simulink model "DC_Microgrid_Sim"  (R2023b)
settings: Solver=VariableStepDiscrete  StartTime=0.0  StopTime=72  MaxStep=1e-2  RelTol=1e-3
undefined symbols (not defined in the file or in its folder): dEgdT, EgRef, gcbh, Ion, k1, Lithium, Rsh_array5pc, sps_rtmsupport, Tref_K, Tsf, VT_ref
libraries: spsSeriesRLCBranchLib x7, spsVoltageMeasurementLib x5, SignalEditorBlockLib x2, spsCurrentMeasurementLib x2, spsDiodeLib x2, spsFirstOrderFilterLib x2, spsControlledCurrentSourceLib x2, spsPVarrayModel x2, spsBatteryLib x1, spsVariableResistorLib x1, spsBoostConverterLib x1, spsStairGeneratorLib x1
(part 9 of 9)

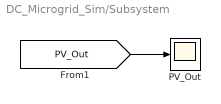
== system DC_Microgrid_Sim/Subsystem ==
  PV_Out : Scope
  wires:
  [PV_Out] -> PV_Out/1

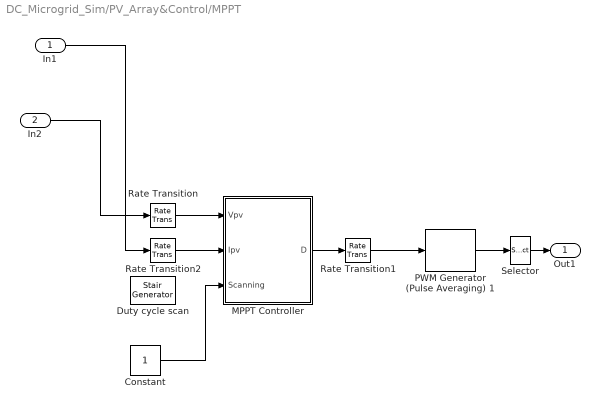
== system DC_Microgrid_Sim/PV_Array&Control/MPPT ==
  In1 : Inport
  In2 : Inport  Port=2
  Constant : Constant
  Duty cycle scan : spsStairGeneratorLib/Stair Generator  t=[0,0.40, 0.41]  e=[0, 1, 0]  Ts=2.5e-05
  MPPT Controller : Subsystem  mask(MPPT Controller - Perturb and Observe algorithm (PandO)){Dinit=0.39, Dlimits=[0.85, 0.30], deltaD=50e-6, Fc=1000, ScanDuration=0.25, Ts=2.5e-05}
      mask prompts: Dinit "Duty cycle (D) initial value"; Dlimits "D limits [Upper, Lower]"; deltaD "Increment value for PandO algorithm"; Fc "Measurement filter cutoff frequency (Hz)"; ScanDuration "Scanning mode duration (s)"; Ts "Sample time (s)"
      mask init:
      | Dmax=Dlimits(1);
      | Dmin=Dlimits(2);
      | SampleTime=Ts;
      | DeltaD_Scan=(Dmax-Dmin)*Ts/ScanDuration;
  PWM Generator (Pulse Averaging) 1 : spsPWMGeneratorPulseAveragingLib/PWM Generator (Pulse Averaging)  GeneratorType=Two-quadrant  Fc=20e3  InitialPhase=90  Ts=5e-06
  Rate Transition : RateTransition  OutPortSampleTime=2.5e-05
  Rate Transition1 : RateTransition  OutPortSampleTime=5e-06
  Rate Transition2 : RateTransition  OutPortSampleTime=2.5e-05
  Selector : Selector  InputPortWidth=2  IndexOptions=Index vector (dialog)  Indices=1  OutputSizes=1
  Out1 : Outport
  wires:
  Selector/1 -> Out1/1
  Rate Transition2/1 -> MPPT Controller/2(Ipv)
  In1/1 -> Rate Transition2/1
  In2/1 -> Rate Transition/1
  Rate Transition1/1 -> PWM Generator (Pulse Averaging) 1/1
  MPPT Controller/1(D) -> Rate Transition1/1
  Rate Transition/1 -> MPPT Controller/1(Vpv)
  PWM Generator (Pulse Averaging) 1/1 -> Selector/1
  Constant/1 -> MPPT Controller/3(Scanning)

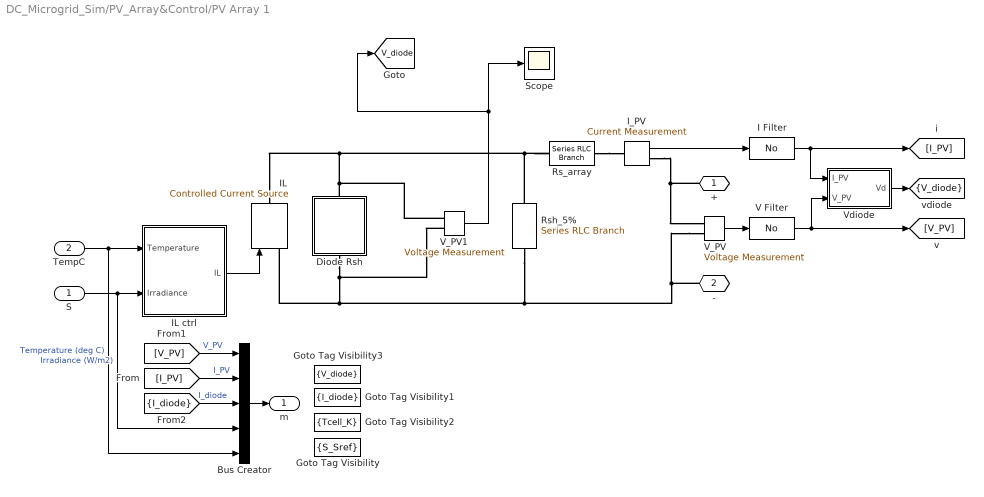
== system DC_Microgrid_Sim/PV_Array&Control/PV Array 1 ==
  S : Inport
  TempC : Inport  Port=2
  Bus Creator : BusCreator  Inputs=5
  Diode Rsh : Subsystem  AncestorBlock=spsPVarrayModel/Discrete Diode Rsh BAL
      mask Display:
      | plot(-75,-50,100,150, [-15 -15 43 -15 -15 -75],[50 8 50 92 50 50], ...
      |     [43 43],[8 94],[100 43], [50 50])
  Goto Tag Visibility : GotoTagVisibility  GotoTag=S_Sref
  Goto Tag Visibility1 : GotoTagVisibility  GotoTag=I_diode
  Goto Tag Visibility2 : GotoTagVisibility  GotoTag=Tcell_K
  Goto Tag Visibility3 : GotoTagVisibility  GotoTag=V_diode
  I Filter : spsPVarrayModel/No  SystemSampleTime=-1  VariantControl=Variant1  VariantActivationTime=update diagram  AllowFlexibleInterface=on  Latency=0  AutoFrameSizeCalculation=off
  IL : spsControlledCurrentSourceLib/Controlled Current Source  Initialize=on  Source_Type=AC  Amplitude=0  Phase=0  Frequency=0  Measurements=None
  IL ctrl : Subsystem
  I_PV : spsCurrentMeasurementLib/Current Measurement  PhasorSimulation=off  OutputType=Complex  PSBequivalent=0
  Rs_array : spsSeriesRLCBranchLib/Series RLC Branch  LConnTagsString=__new0  RConnTagsString=__new0  BranchType=R  Resistance=Rs*Nser/Npar  Inductance=1e-3  SetiL0=off  InitialCurrent=0  Capacitance=1e-6  Setx0=off  InitialVoltage=0  Measurements=None
  Rsh_5% : spsSeriesRLCBranchLib/Series RLC Branch  LConnTagsString=__new0  RConnTagsString=__new0  BranchType=R  Resistance=Rsh_array5pc  Inductance=1e-3  SetiL0=off  InitialCurrent=0  Capacitance=1e-6  Setx0=off  InitialVoltage=0  Measurements=None
  Scope : Scope
  V Filter : spsPVarrayModel/No  SystemSampleTime=-1  VariantControl=Variant1  VariantActivationTime=update diagram  AllowFlexibleInterface=on  Latency=0  AutoFrameSizeCalculation=off
  V_PV : spsVoltageMeasurementLib/Voltage Measurement  PhasorSimulation=off  OutputType=Complex  PSBequivalent=0
  V_PV1 : spsVoltageMeasurementLib/Voltage Measurement  PhasorSimulation=off  OutputType=Complex  PSBequivalent=0
  Vdiode : Subsystem
  + : PMIOPort  Side=Right
  - : PMIOPort  Port=2  Side=Right
  m : Outport  VectorParamsAs1DForOutWhenUnconnected=off
  tag scope: V_diode=global, V_diode=scoped
  wires:
  TempC/1 -> Bus Creator/5, IL ctrl/1(Temperature)  "Temperature (deg C)"
  S/1 -> IL ctrl/2(Irradiance), Bus Creator/4  "Irradiance (W/m2)"
  I_PV/1 -> I Filter/1
  Bus Creator/1 -> m/1
  IL ctrl/1(IL) -> IL/1
  V_PV/1 -> V Filter/1
  I Filter/1 -> Vdiode/1(I_PV), [I_PV]
  V Filter/1 -> [V_PV], Vdiode/2(V_PV)
  [I_PV] -> Bus Creator/2  "I_PV"
  [V_PV] -> Bus Creator/1  "V_PV"
  [I_diode] -> Bus Creator/3  "I_diode"
  Vdiode/1(Vd) -> [V_diode]
  V_PV1/1 -> [V_diode], Scope/1
  connections:
  +/RConn1 -- I_PV/RConn1 -- V_PV/LConn1
  Rs_array/LConn1 -- V_PV1/LConn1 -- Diode Rsh/LConn1 -- IL/RConn1 -- Rsh_5%/LConn1
  V_PV/LConn2 -- V_PV1/LConn2 -- Diode Rsh/RConn1 -- IL/LConn1 -- Rsh_5%/RConn1 -- -/RConn1
  Rs_array/RConn1 -- I_PV/LConn1

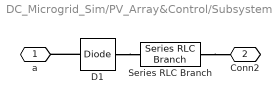
== system DC_Microgrid_Sim/PV_Array&Control/Subsystem ==
  D1 : spsDiodeLib/Diode  Ron=1e-3  Lon=0  Vf=.6  IC=0  UseSnubber=0  Rs=1e6  Cs=inf  Measurements=off
  Series RLC Branch : spsSeriesRLCBranchLib/Series RLC Branch  LConnTagsString=__new0  RConnTagsString=__new0  BranchType=RL  Resistance=20e-3  Inductance=20e-3  SetiL0=off  InitialCurrent=0  Capacitance=1e-6  Setx0=off  InitialVoltage=0  Measurements=None
  a : PMIOPort  Side=Left
  Conn2 : PMIOPort  Port=2  Side=Right
  connections:
  D1/LConn1 -- a/RConn1
  Series RLC Branch/RConn1 -- Conn2/RConn1
  D1/RConn1 -- Series RLC Branch/LConn1

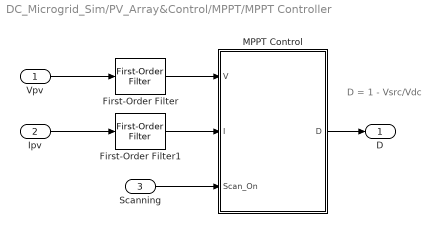
== system DC_Microgrid_Sim/PV_Array&Control/MPPT/MPPT Controller ==
  note: D = 1 - Vsrc/Vdc
  Vpv : Inport
  Ipv : Inport  Port=2
  Scanning : Inport  Port=3  PortDimensions=1
  First-Order Filter : spsFirstOrderFilterLib/First-Order Filter  FilterType=Lowpass  Tc=1/Fc  Ts=Ts  Initialize=off  Vac_Init=[0, 0, 60]  Vdc_Init=0  PlotResponse=off  FreqRange="[0,  200,  1]"
  First-Order Filter1 : spsFirstOrderFilterLib/First-Order Filter  FilterType=Lowpass  Tc=1/Fc  Ts=Ts  Initialize=off  Vac_Init=[0, 0, 60]  Vdc_Init=0  PlotResponse=off  FreqRange="[0,  200,  1]"
  MPPT Control : MATLAB Function  TreatAsAtomicUnit=on
  D : Outport  OutDataTypeStr=double  PortDimensions=1  VectorParamsAs1DForOutWhenUnconnected=off
  wires:
  First-Order Filter1/1 -> MPPT Control/2(I)
  First-Order Filter/1 -> MPPT Control/1(V)
  Ipv/1 -> First-Order Filter1/1
  Vpv/1 -> First-Order Filter/1
  MPPT Control/1(D) -> D/1
  Scanning/1 -> MPPT Control/3(Scan_On)

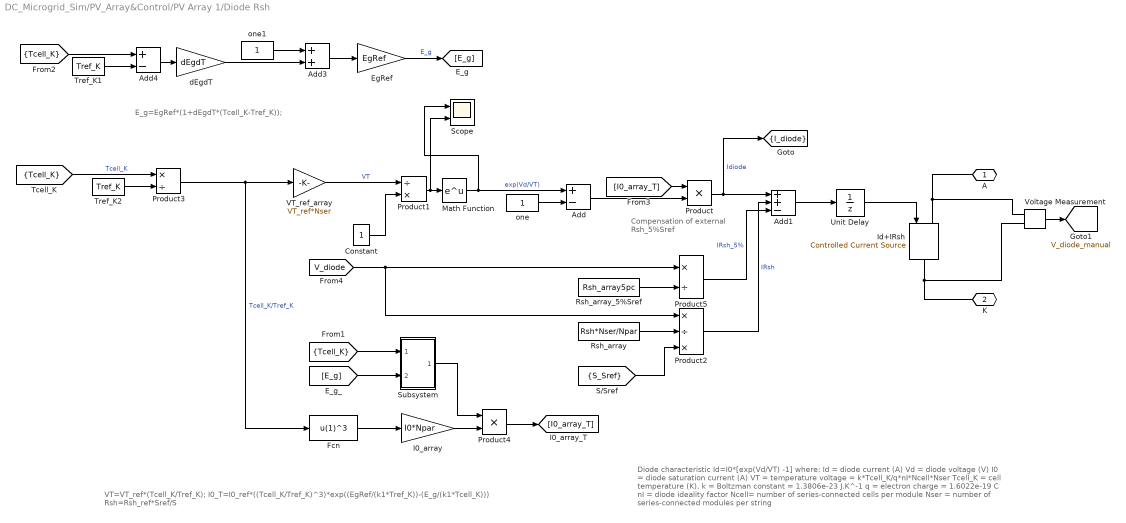
== system DC_Microgrid_Sim/PV_Array&Control/PV Array 1/Diode Rsh ==
  note: E_g=EgRef*(1+dEgdT*(Tcell_K-Tref_K));
  note: VT=VT_ref*(Tcell_K/Tref_K);
      | I0_T=I0_ref*((Tcell_K/Tref_K)^3)*exp((EgRef/(k1*Tref_K))-(E_g/(k1*Tcell_K)))
      | Rsh=Rsh_ref*Sref/S
  note: Diode characteristic
      |    Id=I0*[exp(Vd/VT) -1]
      |
      | where:
      |      Id = diode current (A)
      |      Vd = diode voltage (V)
      |      I0 = diode saturation current (A)
      |      VT = temperature voltage = k*Tcell_K/q*nI*Ncell*Nser
      | Tcell_K = cell temperature (K),
      |       k = Boltzman constant = 1.3806e-23 J.K^-1
      |       q = electron charge = 1.6022e-19 C
      |      nI = diode ideality factor
      |    Ncell= number of series-connected cells per module
      |    Nser = number of series-connected modules per string
  note: Compensation of
      | external Rsh_5%Sref
  Add : Sum  Inputs=+-
  Add1 : Sum  Inputs=++-
  Add3 : Sum
  Add4 : Sum  Inputs=+-
  Constant : Constant
  EgRef : Gain  Gain=EgRef
  Fcn : Fcn  Expr=u(1)^3
  I0_array : Gain  Gain=I0*Npar
  Id+IRsh : spsControlledCurrentSourceLib/Controlled Current Source  Initialize=on  Source_Type=AC  Amplitude=0  Phase=0  Frequency=0  Measurements=None
  Math Function : Math  SignedPower=on
  Product : Product  RndMeth=Zero
  Product1 : Product  Inputs=/*  RndMeth=Zero
  Product2 : Product  Inputs=*/*  RndMeth=Zero
  Product3 : Product  Inputs=*/  RndMeth=Zero
  Product4 : Product  Inputs=**  RndMeth=Zero
  Product5 : Product  Inputs=*/  RndMeth=Zero
  Rsh_array : Constant  Value=Rsh*Nser/Npar
  Rsh_array_5%Sref : Constant  Value=Rsh_array5pc
  Scope : Scope  NumInputPorts=2
  Subsystem : Subsystem
  Tref_K1 : Constant  Value=Tref_K
  Tref_K2 : Constant  Value=Tref_K
  Unit Delay : UnitDelay  SampleTime=Tsf  HasFrameUpgradeWarning=on
  VT_ref_array : Gain  Gain=VT_ref*Nser
  Voltage Measurement : spsVoltageMeasurementLib/Voltage Measurement  PhasorSimulation=off  OutputType=Complex  PSBequivalent=0
  dEgdT : Gain  Gain=dEgdT
  one : Constant
  one1 : Constant
  A : PMIOPort  Side=Left
  K : PMIOPort  Port=2  Side=Right
  tag scope: I_diode=scoped, V_diode_manual=global
  wires:
  [V_diode] -> Product2/1, Product5/1
  [S_Sref] -> Product2/3
  [I0_array_T] -> Product/1
  VT_ref_array/1 -> Product1/1  "VT"
  Add/1 -> Product/2
  Product4/1 -> [I0_array_T]
  Tref_K2/1 -> Product3/2
  [E_g] -> Subsystem/2(E_g)
  [Tcell_K] -> Subsystem/1(Tcell_K)
  Subsystem/1(exp) -> Product4/1
  Tref_K1/1 -> Add4/2
  [Tcell_K] -> Add4/1
  Fcn/1 -> I0_array/1
  I0_array/1 -> Product4/2
  EgRef/1 -> [E_g]  "E_g"
  Add3/1 -> EgRef/1
  dEgdT/1 -> Add3/2
  Add4/1 -> dEgdT/1
  one1/1 -> Add3/1
  Product3/1 -> Fcn/1, VT_ref_array/1  "Tcell_K/Tref_K"
  [Tcell_K] -> Product3/1  "Tcell_K"
  Rsh_array/1 -> Product2/2
  one/1 -> Add/2
  Product1/1 -> Scope/2, Math Function/1
  Product/1 -> [I_diode], Add1/1  "Idiode"
  Product2/1 -> Add1/2  "IRsh"
  Math Function/1 -> Scope/1, Add/1  "exp(Vd/VT)"
  Rsh_array_5%Sref/1 -> Product5/2
  Product5/1 -> Add1/3  "IRsh_5%"
  Add1/1 -> Unit Delay/1
  Unit Delay/1 -> Id+IRsh/1
  Voltage Measurement/1 -> [V_diode_manual]
  Constant/1 -> Product1/2
  connections:
  A/RConn1 -- Id+IRsh/LConn1 -- Voltage Measurement/LConn1
  Id+IRsh/RConn1 -- Voltage Measurement/LConn2 -- K/RConn1

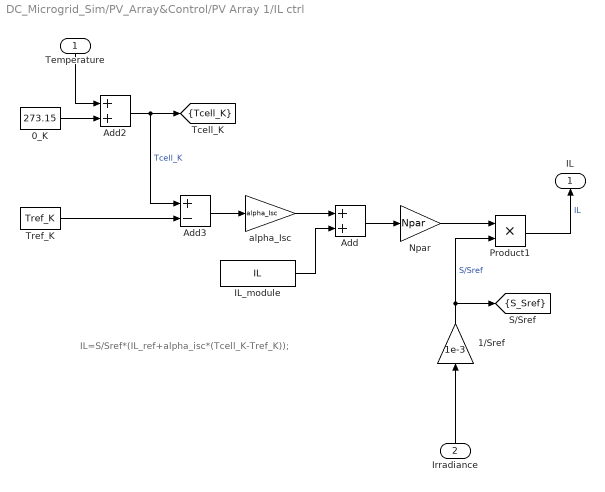
== system DC_Microgrid_Sim/PV_Array&Control/PV Array 1/IL ctrl ==
  note: IL=S/Sref*(IL_ref+alpha_isc*(Tcell_K-Tref_K));
  Temperature : Inport
  Irradiance : Inport  Port=2
  0_K : Constant  Value=273.15
  1/Sref : Gain  Gain=1e-3
  Add : Sum
  Add2 : Sum
  Add3 : Sum  Inputs=+-
  IL_module : Constant  Value=IL
  Npar : Gain  Gain=Npar
  Product1 : Product  Inputs=**  RndMeth=Zero
  Tref_K : Constant  Value=Tref_K
  alpha_Isc : Gain  Gain=alpha_Isc
  IL : Outport  VectorParamsAs1DForOutWhenUnconnected=off
  tag scope: S_Sref=scoped, Tcell_K=scoped
  wires:
  1/Sref/1 -> [S_Sref], Product1/2  "S/Sref"
  Npar/1 -> Product1/1
  Add2/1 -> [Tcell_K], Add3/1  "Tcell_K"
  Add/1 -> Npar/1
  0_K/1 -> Add2/2
  IL_module/1 -> Add/2
  Product1/1 -> IL/1  "IL"
  Tref_K/1 -> Add3/2
  Add3/1 -> alpha_Isc/1
  alpha_Isc/1 -> Add/1
  Irradiance/1 -> 1/Sref/1
  Temperature/1 -> Add2/1

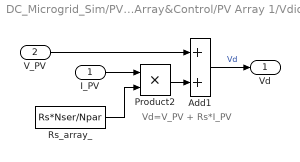
== system DC_Microgrid_Sim/PV_Array&Control/PV Array 1/Vdiode ==
  note: Vd=V_PV + Rs*I_PV
  I_PV : Inport
  V_PV : Inport  Port=2
  Add1 : Sum
  Product2 : Product  Inputs=**  RndMeth=Zero
  Rs_array_ : Constant  Value=Rs*Nser/Npar
  Vd : Outport  VectorParamsAs1DForOutWhenUnconnected=off
  wires:
  Add1/1 -> Vd/1  "Vd"
  I_PV/1 -> Product2/1
  Product2/1 -> Add1/2
  V_PV/1 -> Add1/1
  Rs_array_/1 -> Product2/2

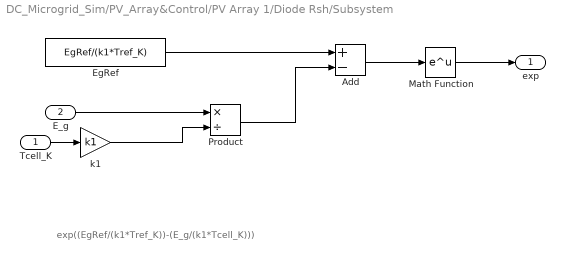
== system DC_Microgrid_Sim/PV_Array&Control/PV Array 1/Diode Rsh/Subsystem ==
  note: exp((EgRef/(k1*Tref_K))-(E_g/(k1*Tcell_K)))
  Tcell_K : Inport
  E_g : Inport  Port=2
  Add : Sum  Inputs=+-
  EgRef : Constant  Value=EgRef/(k1*Tref_K)
  Math Function : Math  SignedPower=on
  Product : Product  Inputs=*/
  k1 : Gain  Gain=k1
  exp : Outport  VectorParamsAs1DForOutWhenUnconnected=off
  wires:
  Math Function/1 -> exp/1
  Add/1 -> Math Function/1
  Product/1 -> Add/2
  k1/1 -> Product/2
  Tcell_K/1 -> k1/1
  E_g/1 -> Product/1
  EgRef/1 -> Add/1

== matlab function DC_Microgrid_Sim/PV_Array&Control/MPPT/MPPT Controller/MPPT Control ==
  settings: updateMethod=DISCRETE  sampleTime=Ts
  data: V input =V; I input; D output; Dmax parameter; Dmin parameter; deltaD parameter; Dinit parameter; Scan_On input; DeltaD_Scan parameter
function D   = PandO(V, I, Dmax, Dmin, deltaD, Dinit, Scan_On, DeltaD_Scan)

% MPPT controller based on the Perturb & Observe algorithm.

% D output = Duty cycle of the boost converter (value between 0 and 1)
% V input = PV array terminal voltage (V)
% I input = PV array current (A)
% D = 1 - Vinput/Voutput (increasing D decrease Vin)

persistent Vold Pold Dold Scan_On_Old Pmax D_Pmax V_Pmax;
%
if isempty(Vold)
    Vold=0;
    Pold=0;
    Scan_On_Old=0;
    Dold=Dinit;
    Pmax=0;
    D_Pmax=0;
    V_Pmax=0;
end
P= V*I;
if Scan_On==1 || Scan_On_Old==1
    if Scan_On_Old==0
        Scan_On_Old=1;
        D=Dmin;
    else
        D=Dold+DeltaD_Scan;
    end
    Dold=D;
    if P>Pmax
        Pmax=P;
        D_Pmax=D;
    end
    if D >= Dmax
        Scan_On_Old=0;
        Pold=Pmax;
        Dold=D_Pmax;
        Vold=V_Pmax;
    end
else
    dV= V - Vold;
    dP= P - Pold;
    %
    if dP ~= 0
        if dP < 0
            if dV < 0
                D = Dold - deltaD;
            else
                D = Dold + deltaD;
            end
        else
            if dV < 0
                D = Dold + deltaD;
            else
                D = Dold - deltaD;
            end
        end
    else
        D=Dold;
    end
    %
    if D >= Dmax || D<= Dmin
        D=Dold;
    end
    %
    Dold=D;
    Vold=V;
    Pold=P;
end

== matlab function DC_Microgrid_Sim/Load_Sim/MATLAB Function ==
  data: power input; resistance output; voltage input
function resistance = fcn(power,voltage)

resistance = (voltage^2)/power;
